simulink model "validation"  (R2017b)
settings: Solver=ode8  StartTime=0.0  StopTime=time_sim  FixedStep=1/Fs  MaxStep=1e-4  RelTol=1e-3  EnableMultiTasking=on
values from neighbouring files (symbols this model uses):
  beta = Y(n,5)    [datos_entrenamiento.m]    (also in hiperparametros.m = ypred(5); prediccion.m = round(beta*100,2); sensibilidad.m = ypred(5))
  f = 50    [hiperparametros.m]    (also in prediccion.m; sensibilidad.m)
  Fs = 4*Fm; save([PathFolder '/Fs'],'Fs')    [datos_entrenamiento.m]    (also in prediccion.m = 4*Fm; sensibilidad.m = 4*Fm)
  k1 = Y(n,1)    [datos_entrenamiento.m]    (also in hiperparametros.m = ypred(1); prediccion.m = round(k1*10000,2); sensibilidad.m = ypred(1))
  k2 = Y(n,2)    [datos_entrenamiento.m]    (also in hiperparametros.m = ypred(2); prediccion.m = round(k2*10,2); sensibilidad.m = ypred(2))
  k3 = Y(n,3)    [datos_entrenamiento.m]    (also in hiperparametros.m = ypred(3); prediccion.m = round(k3*15,2); sensibilidad.m = ypred(3))
  Lc = Y(n,8)    [datos_entrenamiento.m]    (also in hiperparametros.m = ypred(8); prediccion.m = Lc*0.00001; sensibilidad.m = ypred(8))
  Leaf_pu = 0.1    [prediccion.m]    (also in sensibilidad.m)
  Lt1_pu = 0.12    [prediccion.m]    (also in sensibilidad.m)
  Rc = Y(n,7)    [datos_entrenamiento.m]    (also in hiperparametros.m = ypred(7); prediccion.m = Rc*0.001; sensibilidad.m = ypred(7))
  Reaf_pu = 0.01    [prediccion.m]    (also in sensibilidad.m)
  Rt1_pu = 0.012    [prediccion.m]    (also in sensibilidad.m)
  Rthe = 1.9    [prediccion.m]    (also in sensibilidad.m)
  s = Y(n,4)    [datos_entrenamiento.m]    (also in hiperparametros.m = ypred(4); prediccion.m = round(s*100,2); sensibilidad.m = ypred(4))
  Seaf = 30e6    (= 30000000)    [prediccion.m]    (also in sensibilidad.m)
  St1 = 42e6    (= 42000000)    [prediccion.m]    (also in sensibilidad.m)
  V1eaf = 11000    [prediccion.m]    (also in sensibilidad.m)
  V1t1 = 115000    [prediccion.m]    (also in sensibilidad.m)
  V2eaf = 760    [prediccion.m]    (also in sensibilidad.m)
  V2t1 = 11000    [prediccion.m]    (also in sensibilidad.m)
  w = Y(n,6)    [datos_entrenamiento.m]    (also in hiperparametros.m = ypred(6); prediccion.m = round(w*1,2); sensibilidad.m = ypred(6))
  Xthe = 5*37.7    (= 188.5)    [prediccion.m]    (also in sensibilidad.m)
  Zsec = 1e-6    (= 1e-06)    [prediccion.m]    (also in sensibilidad.m)
libraries: powerlib x19, powerlib_meascontrol x2
PreSaveFcn:
  | RO=12.5;
  | L=3.6;
  | C1=0.000002;
  | C2=0.000020;
  | G=0.0005442;
  | 
  | I30=-1.810e-3;
  | V10=2.286;
  | V20=-222.014e-3;
  | 
  | E=1;
  | Ga=-757.576e-6;
  | Gb=-409.091e-6;
  | 
  | r0=10;
  | k1=3000;
  | k2=1.0;
  | k3=12.5;
  | 
  | m=0;
  | n=2;
settings Model: Creator=Administrador  LastModifiedBy=Jesser
settings DataIOCC: SaveFormat=Array  SignalLoggingSaveFormat=ModelDataLogs  TimeSaveName=t
settings OptimizationCC: ExpressionDepthLimit=2147483647  InitFltsAndDblsToZero=on  LifeSpan=inf
settings DebuggingCC: SaveWithParameterizedLinksMsg=none  UnderspecifiedInitializationDetection=Classic  MergeDetectMultiDrivingBlocksExec=none  SolverPrmCheckMsg=warning  FcnCallInpInsideContextMsg=warning  StateNameClashWarn=warning  StrictBusMsg=Warning  SFUnexpectedBacktrackingDiag=warning  SFNoUnconditionalDefaultTransitionDiag=warning  SFExecutionAtInitializationDiag=none
settings HardwareCC: ProdBitPerPointer=32  ProdBitPerSizeT=32  ProdBitPerPtrDiffT=32  ProdLargestAtomicFloat=None  ProdIntDivRoundTo=Undefined  ProdEndianess=Unspecified  ProdWordSize=32  ProdHWDeviceType=32-bit Generic
settings ModelReferenceCC: PropagateSignalLabelsOutOfModel=off
settings CodeAppCC: StateflowObjectComments=on
settings GRTTargetCC: TargetLangStandard=C89/C90 (ANSI)  CombineOutputUpdateFcns=off  GRTInterface=on
settings ConfigComp: CovMetricSettings=dw  CovHtmlReporting=on  CovSaveCumulativeToWorkspaceVar=on  CovSaveSingleToWorkspaceVar=on  CovExternalEMLEnable=off

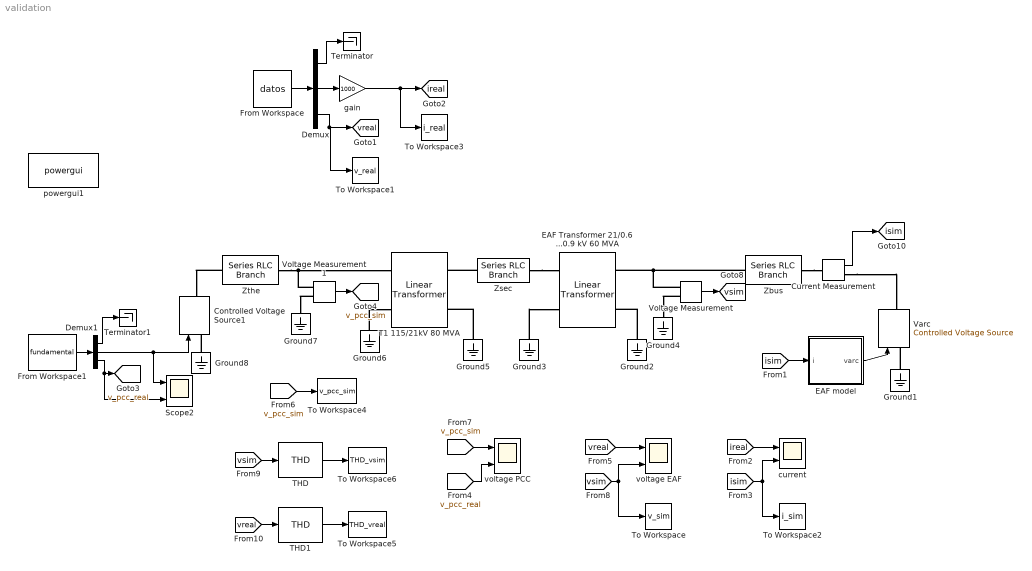
== system validation ==
  Controlled Voltage Source1 : powerlib/Electrical Sources/Controlled Voltage Source  Initialize=off  Source_Type=AC  Amplitude=0  Phase=0  Frequency=0  Measurements=None
  Current Measurement : powerlib/Measurements/Current Measurement  PhasorSimulation=off  OutputType=Complex  PSBequivalent=0
  Demux : Demux  Outputs=3
  Demux1 : Demux  Outputs=3
  EAF Transformer 21/0.6 ...0.9 kV 60 MVA : powerlib/Elements/Linear Transformer  UNITS=pu  NominalPower=[Seaf/3 f]  winding1=[V1eaf Reaf_pu Leaf_pu]  winding2=[V2eaf 1e-7 1e-6]  ThreeWindings=off  winding3=[3.15e+05 0.00025333 0.010133]  RmLm=[50000 50000]  Measurements=None  DataType=off
  EAF model : Subsystem
  From Workspace : FromWorkspace  VariableName=datos  SampleTime=0
  From Workspace1 : FromWorkspace  VariableName=fundamental  SampleTime=0
  Ground{1..8} (8 alike) : powerlib/Elements/Ground  LConnTagsString=a
  Scope2 : Scope  NumInputPorts=2
  T1 115/21kV 80 MVA : powerlib/Elements/Linear Transformer  UNITS=pu  NominalPower=[St1/3 f]  winding1=[V1t1 Rt1_pu Lt1_pu]  winding2=[V2t1 1e-6 1e-5]  ThreeWindings=off  winding3=[3.15e+05 0.00025333 0.010133]  RmLm=[50000 50000]  Measurements=None  DataType=off
  THD : powerlib_meascontrol/Measurements/THD  Freq=50  Ts=0
  THD1 : powerlib_meascontrol/Measurements/THD  Freq=50  Ts=0
  Terminator : Terminator
  Terminator1 : Terminator
  To Workspace : ToWorkspace  VariableName=v_sim  SampleTime=-1
  To Workspace1 : ToWorkspace  VariableName=v_real  SampleTime=-1
  To Workspace2 : ToWorkspace  VariableName=i_sim  SampleTime=-1
  To Workspace3 : ToWorkspace  VariableName=i_real  SampleTime=-1
  To Workspace4 : ToWorkspace  VariableName=v_pcc_sim  SampleTime=-1
  To Workspace5 : ToWorkspace  VariableName=THD_vreal  SampleTime=-1
  To Workspace6 : ToWorkspace  VariableName=THD_vsim  SampleTime=-1
  Varc : powerlib/Electrical Sources/Controlled Voltage Source  Initialize=off  Source_Type=AC  Amplitude=0  Phase=0  Frequency=0  Measurements=None
  Voltage Measurement : powerlib/Measurements/Voltage Measurement  PhasorSimulation=off  OutputType=Complex  PSBequivalent=0
  Voltage Measurement1 : powerlib/Measurements/Voltage Measurement  PhasorSimulation=off  OutputType=Complex  PSBequivalent=0
  Zbus : powerlib/Elements/Series RLC Branch  LConnTagsString=__new0  RConnTagsString=__new0  BranchType=RL  Resistance=Rc*1e-3  Inductance=Lc*1e-5  SetiL0=off  InitialCurrent=0  Capacitance=1e-6  Setx0=off  InitialVoltage=0  Measurements=None
  Zsec : powerlib/Elements/Series RLC Branch  LConnTagsString=__new0  RConnTagsString=__new0  BranchType=L  Resistance=1.9  Inductance=Zsec/(2*pi*f)  SetiL0=off  InitialCurrent=0  Capacitance=1e-6  Setx0=off  InitialVoltage=0  Measurements=None
  Zthe : powerlib/Elements/Series RLC Branch  LConnTagsString=__new0  RConnTagsString=__new0  BranchType=RL  Resistance=Rthe  Inductance=Xthe/(2*pi*f)  SetiL0=off  InitialCurrent=0  Capacitance=1e-6  Setx0=off  InitialVoltage=0  Measurements=None
  current : Scope  NumInputPorts=2
  gain : Gain  Gain=1000
  powergui1 : powerlib/powergui  Priority=1  SimulationMode=Discrete  SampleTime=1/Fs  frequency=60  Iterations=50  frequencyindice=0  Pbase=100e6  ErrMax=1e-4  UnitsV=kV  UnitsW=MW  buscounter=0  FunctionMessages=off  echomessages=off  EnableUseOfTLC=off  CurrentSourceSwitches=off  DisableSnubberDevices=off  DisableRonSwitches=off  DisableVfSwitches=off  DisplayEquations=off  SolverType=Tustin/Backward Euler (TBE)  Interpol=off  ExternalGateDelay=off  methode=off  Ts=100  x0status=blocks  SPID=off  SwTol=0  HookPort=off  RestoreLinks=warning  ResistiveCurrentMeasurement=off  Frange=[0:2:500]  Ylog=off  Xlog=on  ShowGrid=off  save=off  variable=ZData  structure=0  ZoomFFT=off  StartTime=0.0  cycles=1  DisplayStyle=1  fundamental=60  FreqAxis=off  MaxFrequency=1000  frequencyindicesteady=1  RmsSteady=1  display=off
  voltage EAF : Scope  NumInputPorts=2
  voltage PCC : Scope  NumInputPorts=2
  tag scope: ireal=global, isim=global, v_pcc_real=global, v_pcc_sim=global, vreal=global, vsim=global
  wires:
  From Workspace/1 -> Demux/1
  Demux/1 -> Terminator/1
  Demux/3 -> To Workspace1/1, [vreal]
  [vreal] -> voltage EAF/1
  Current Measurement/1 -> [isim]
  EAF model/1(varc) -> Varc/1
  Voltage Measurement/1 -> [vsim]
  [vsim] -> To Workspace/1, voltage EAF/2
  [isim] -> EAF model/1(i)
  [ireal] -> current/1
  [isim] -> To Workspace2/1, current/2
  From Workspace1/1 -> Demux1/1
  Demux1/1 -> Terminator1/1
  Demux1/2 -> Scope2/1, Controlled Voltage Source1/1
  Demux/2 -> gain/1
  gain/1 -> To Workspace3/1, [ireal]
  Demux1/3 -> Scope2/2, [v_pcc_real]
  [v_pcc_real] -> voltage PCC/2
  Voltage Measurement1/1 -> [v_pcc_sim]
  [v_pcc_sim] -> To Workspace4/1
  [v_pcc_sim] -> voltage PCC/1
  [vsim] -> THD/1
  [vreal] -> THD1/1
  THD/1 -> To Workspace6/1
  THD1/1 -> To Workspace5/1
  connections:
  Ground8/LConn1 -- Controlled Voltage Source1/LConn1
  Ground1/LConn1 -- Varc/LConn1
  Ground2/LConn1 -- EAF Transformer 21/0.6 ...0.9 kV 60 MVA/RConn2
  Ground3/LConn1 -- EAF Transformer 21/0.6 ...0.9 kV 60 MVA/LConn2
  Zbus/RConn1 -- Current Measurement/LConn1
  Current Measurement/RConn1 -- Varc/RConn1
  Zbus/LConn1 -- Voltage Measurement/LConn1 -- EAF Transformer 21/0.6 ...0.9 kV 60 MVA/RConn1
  Voltage Measurement/LConn2 -- Ground4/LConn1
  Ground5/LConn1 -- T1 115/21kV 80 MVA/RConn2
  Ground6/LConn1 -- T1 115/21kV 80 MVA/LConn2
  Zsec/RConn1 -- EAF Transformer 21/0.6 ...0.9 kV 60 MVA/LConn1
  Zsec/LConn1 -- T1 115/21kV 80 MVA/RConn1
  Zthe/RConn1 -- Voltage Measurement1/LConn1 -- T1 115/21kV 80 MVA/LConn1
  Zthe/LConn1 -- Controlled Voltage Source1/RConn1
  Voltage Measurement1/LConn2 -- Ground7/LConn1

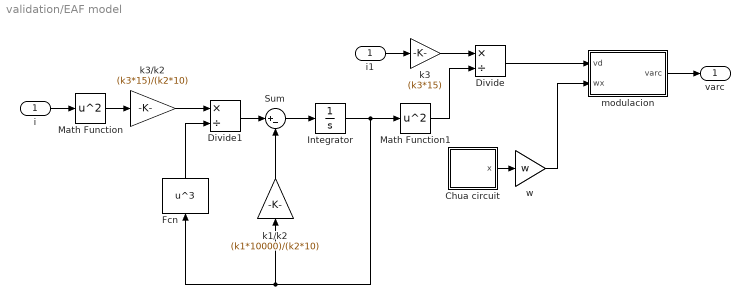
== system validation/EAF model ==
  i : Inport
  "Chua circuit " : Subsystem
  Divide : Product  Inputs=*/
  Divide1 : Product  Inputs=*/
  Fcn : Fcn  Expr=u^3
  Integrator : Integrator  InitialCondition=1e-0
  Math Function : Math  Operator=square  SaturateOnIntegerOverflow=on
  Math Function1 : Math  Operator=square  SaturateOnIntegerOverflow=on
  Sum : Sum  Inputs=|+-
  i1 : InportShadow
  k1/k2 : Gain  Gain=(k1*10000)/(k2*10)
  k3 : Gain  Gain=(k3*15)
  k3/k2 : Gain  Gain=(k3*15)/(k2*10)
  modulacion : Subsystem
  w : Gain  Gain=w
  varc : Outport
  wires:
  Math Function/1 -> k3/k2/1
  Fcn/1 -> Divide1/2
  Divide1/1 -> Sum/1
  k1/k2/1 -> Sum/2
  Sum/1 -> Integrator/1
  k3/k2/1 -> Divide1/1
  k3/1 -> Divide/1
  Math Function1/1 -> Divide/2
  i/1 -> Math Function/1
  i1/1 -> k3/1
  Integrator/1 -> Math Function1/1, Fcn/1, k1/k2/1
  Divide/1 -> modulacion/1(vd)
  modulacion/1(varc) -> varc/1
  "Chua circuit "/1(x) -> w/1
  w/1 -> modulacion/2(wx)

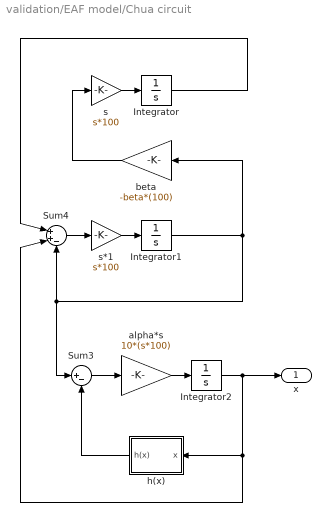
== system validation/EAF model/Chua circuit  ==
  Integrator : Integrator
  Integrator1 : Integrator
  Integrator2 : Integrator  InitialCondition=1
  Sum3 : Sum  Inputs=|+-
  Sum4 : Sum  Inputs=|++-
  alpha*s : Gain  Gain=10*(s*100)
  beta : Gain  Gain=-beta*(100)
  h(x) : Subsystem
  s : Gain  Gain=s*100
  s*1 : Gain  Gain=s*100
  x : Outport
  wires:
  Integrator2/1 -> Sum4/2, h(x)/1(x), x/1
  h(x)/1(h(x)) -> Sum3/2
  Integrator/1 -> Sum4/1
  Integrator1/1 -> Sum3/1, Sum4/3, beta/1
  alpha*s/1 -> Integrator2/1
  Sum3/1 -> alpha*s/1
  beta/1 -> s/1
  s/1 -> Integrator/1
  Sum4/1 -> s*1/1
  s*1/1 -> Integrator1/1

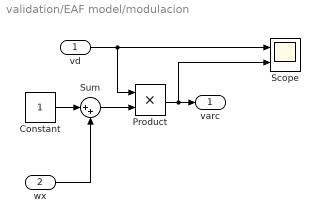
== system validation/EAF model/modulacion ==
  vd : Inport
  wx : Inport  Port=2
  Constant : Constant
  Product : Product
  Scope : Scope  NumInputPorts=2
  Sum : Sum  Inputs=|++
  varc : Outport
  wires:
  wx/1 -> Sum/2
  Constant/1 -> Sum/1
  Product/1 -> Scope/2, varc/1
  vd/1 -> Scope/1, Product/1
  Sum/1 -> Product/2

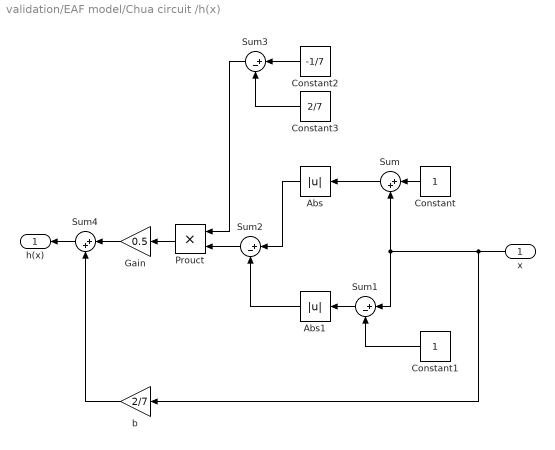
== system validation/EAF model/Chua circuit /h(x) ==
  x : Inport
  Abs : Abs
  Abs1 : Abs
  Constant : Constant
  Constant1 : Constant
  Constant2 : Constant  Value=-1/7
  Constant3 : Constant  Value=2/7
  Gain : Gain  Gain=0.5
  Prouct : Product  RndMeth=Zero
  Sum : Sum  Inputs=|++
  Sum1 : Sum  Inputs=|+-
  Sum2 : Sum  Inputs=|+-
  Sum3 : Sum  Inputs=|+-
  Sum4 : Sum  Inputs=|++
  b : Gain  Gain=2/7
  h(x) : Outport
  wires:
  x/1 -> Sum/2, Sum1/1, b/1
  Constant/1 -> Sum/1
  Constant1/1 -> Sum1/2
  Sum/1 -> Abs/1
  Sum1/1 -> Abs1/1
  Abs/1 -> Sum2/1
  Abs1/1 -> Sum2/2
  Sum2/1 -> Prouct/2
  Constant2/1 -> Sum3/1
  Constant3/1 -> Sum3/2
  Sum3/1 -> Prouct/1
  Prouct/1 -> Gain/1
  Gain/1 -> Sum4/1
  b/1 -> Sum4/2
  Sum4/1 -> h(x)/1
